simulink model "phase_comp_rate_limiter"  (R2016b)
settings: Solver=VariableStepAuto  StartTime=0.0  StopTime=10.0  RelTol=1e-3
settings Model: Creator=nicol  LastModifiedBy=nicol

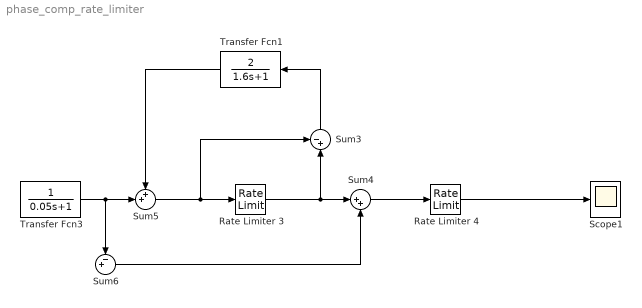
== system phase_comp_rate_limiter ==
  Rate Limiter 3 : RateLimiter  RisingSlewLimit=9.57  FallingSlewLimit=-9.57  SampleTimeMode=inherited
  Rate Limiter 4 : RateLimiter  RisingSlewLimit=9.57  FallingSlewLimit=-9.57  SampleTimeMode=inherited
  Scope1 : Scope
  Sum3 : Sum  Inputs=-+|
  Sum4 : Sum  Inputs=|++
  Sum5 : Sum  Inputs=++|
  Sum6 : Sum  Inputs=-+|
  Transfer Fcn1 : TransferFcn  Numerator=[2]  Denominator=[1.6 1]
  Transfer Fcn3 : TransferFcn  Denominator=[0.05 1]
  wires:
  ? -> Transfer Fcn3/1, Sum6/2
  Sum6/1 -> Sum4/2
  Sum4/1 -> Rate Limiter 4/1
  Rate Limiter 3/1 -> Sum3/2, Sum4/1
  Transfer Fcn3/1 -> Sum5/2, Sum6/1
  Sum5/1 -> Sum3/1, Rate Limiter 3/1
  Sum3/1 -> Transfer Fcn1/1
  Transfer Fcn1/1 -> Sum5/1
  Rate Limiter 4/1 -> Scope1/1
